simulink model "ssc_vent_splitter_electrical_seriesbag_arch"  (R2020a)
settings: Solver=VariableStepAuto  StartTime=0.0  StopTime=10.0  RelTol=1e-3
settings Model: Creator=jsolislemus  LastModifiedBy=jsolislemus

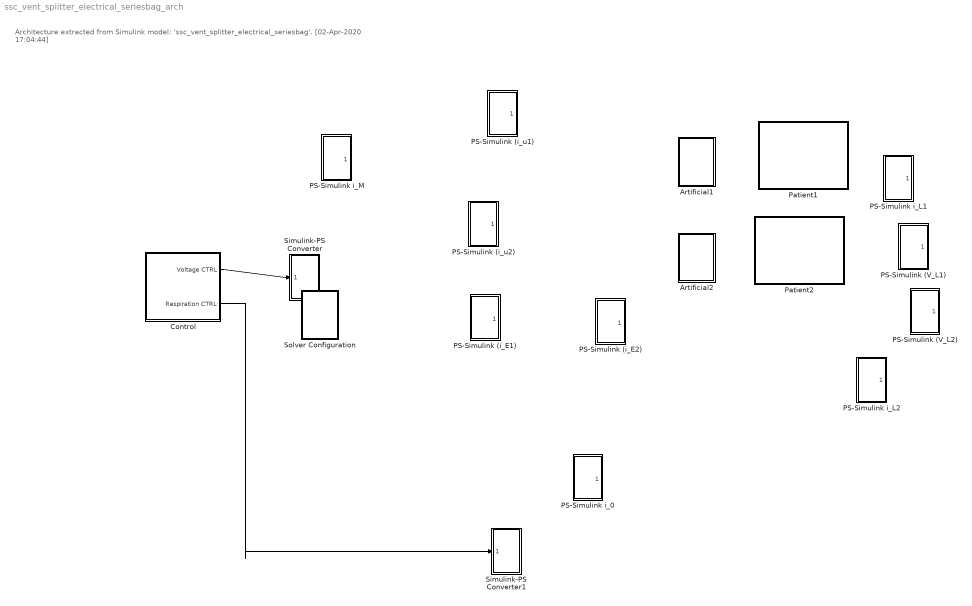
== system ssc_vent_splitter_electrical_seriesbag_arch ==
  note: Architecture extracted from Simulink model: 'ssc_vent_splitter_electrical_seriesbag'. [02-Apr-2020 17:04:44]
  Artificial1 : Subsystem
      settings: PortSchema="{\"entries\":[{\"content\":{\"headerSize\":26,\"margin\":15,\"minimumSpacing\":25,\"sides\":[{\"content\":{\"connectorIds\":[]},\"type\":\"ConnectorPlacement.EquallySpacedRectSide\",\"uuid\":\"6e29aa07-6d05-406a-a3ec-411c5a5a6d59\"},{\"content\":{\"connectorIds\":[],\"side\":\"RIGHT\"},\"type\":\"ConnectorPlacement.EquallySpacedRectSide\",\"uuid\":\"880d3d42-795d-48a8-b736-07df68c99583\"},{\"content\":{\"connectorIds\":[],\"side\":\"TOP\"},\"type\":\"ConnectorPlacement.EquallySpacedRectSide\",\"uuid\":\"00af69ac-1a44-4698-9ec4-d9939426b1cd\"}]},\"type\":\"ConnectorPlacement.EquallySpacedConnector\",\"uuid\":\"8adbbd94-ea7f-44e1-905b-8cd3d9e7fadd\"}],\"packageUris\":[\"http://schema.mathworks.com/mf0/Connector/19700101\"],\"version\":\"1.0\"}"
  Artificial2 : Subsystem
      settings: PortSchema="{\"entries\":[{\"content\":{\"headerSize\":26,\"margin\":15,\"minimumSpacing\":25,\"sides\":[{\"content\":{\"connectorIds\":[]},\"type\":\"ConnectorPlacement.EquallySpacedRectSide\",\"uuid\":\"6e29aa07-6d05-406a-a3ec-411c5a5a6d59\"},{\"content\":{\"connectorIds\":[],\"side\":\"RIGHT\"},\"type\":\"ConnectorPlacement.EquallySpacedRectSide\",\"uuid\":\"880d3d42-795d-48a8-b736-07df68c99583\"},{\"content\":{\"connectorIds\":[],\"side\":\"TOP\"},\"type\":\"ConnectorPlacement.EquallySpacedRectSide\",\"uuid\":\"00af69ac-1a44-4698-9ec4-d9939426b1cd\"}]},\"type\":\"ConnectorPlacement.EquallySpacedConnector\",\"uuid\":\"8adbbd94-ea7f-44e1-905b-8cd3d9e7fadd\"}],\"packageUris\":[\"http://schema.mathworks.com/mf0/Connector/19700101\"],\"version\":\"1.0\"}"
  Control : Subsystem
      settings: PortSchema="{\"entries\":[{\"content\":{\"headerSize\":26,\"margin\":15,\"minimumSpacing\":25,\"sides\":[{\"content\":{\"connectorIds\":[]},\"type\":\"ConnectorPlacement.EquallySpacedRectSide\",\"uuid\":\"868cd02f-3873-4bc0-ad03-13679f5ae2c1\"},{\"content\":{\"connectorIds\":[\"Out1\",\"Out2\"],\"side\":\"RIGHT\"},\"type\":\"ConnectorPlacement.EquallySpacedRectSide\",\"uuid\":\"69928d49-2df3-460f-9e90-f50f969c914b\"},{\"content\":{\"connectorIds\":[],\"side\":\"TOP\"},\"type\":\"ConnectorPlacement.EquallySpacedRectSide\",\"uuid\":\"e58060e5-3c0a-4db3-b34f-65b9832dbc59\"}]},\"type\":\"ConnectorPlacement.EquallySpacedConnector\",\"uuid\":\"a075824f-9c8d-4394-bddd-e7a18dd1991b\"}],\"packageUris\":[\"http://schema.mathworks.com/mf0/Connector/19700101\"],\"version\":\"1.0\"}"
  PS-Simulink (V_L1) : Subsystem
      settings: PortSchema="{\"entries\":[{\"content\":{\"headerSize\":26,\"margin\":15,\"minimumSpacing\":25,\"sides\":[{\"content\":{\"connectorIds\":[]},\"type\":\"ConnectorPlacement.EquallySpacedRectSide\",\"uuid\":\"868cd02f-3873-4bc0-ad03-13679f5ae2c1\"},{\"content\":{\"connectorIds\":[\"Out1\"],\"side\":\"RIGHT\"},\"type\":\"ConnectorPlacement.EquallySpacedRectSide\",\"uuid\":\"69928d49-2df3-460f-9e90-f50f969c914b\"},{\"content\":{\"connectorIds\":[],\"side\":\"TOP\"},\"type\":\"ConnectorPlacement.EquallySpacedRectSide\",\"uuid\":\"e58060e5-3c0a-4db3-b34f-65b9832dbc59\"}]},\"type\":\"ConnectorPlacement.EquallySpacedConnector\",\"uuid\":\"a075824f-9c8d-4394-bddd-e7a18dd1991b\"}],\"packageUris\":[\"http://schema.mathworks.com/mf0/Connector/19700101\"],\"version\":\"1.0\"}"
  PS-Simulink (V_L2) : Subsystem
      settings: PortSchema="{\"entries\":[{\"content\":{\"headerSize\":26,\"margin\":15,\"minimumSpacing\":25,\"sides\":[{\"content\":{\"connectorIds\":[]},\"type\":\"ConnectorPlacement.EquallySpacedRectSide\",\"uuid\":\"868cd02f-3873-4bc0-ad03-13679f5ae2c1\"},{\"content\":{\"connectorIds\":[\"Out1\"],\"side\":\"RIGHT\"},\"type\":\"ConnectorPlacement.EquallySpacedRectSide\",\"uuid\":\"69928d49-2df3-460f-9e90-f50f969c914b\"},{\"content\":{\"connectorIds\":[],\"side\":\"TOP\"},\"type\":\"ConnectorPlacement.EquallySpacedRectSide\",\"uuid\":\"e58060e5-3c0a-4db3-b34f-65b9832dbc59\"}]},\"type\":\"ConnectorPlacement.EquallySpacedConnector\",\"uuid\":\"a075824f-9c8d-4394-bddd-e7a18dd1991b\"}],\"packageUris\":[\"http://schema.mathworks.com/mf0/Connector/19700101\"],\"version\":\"1.0\"}"
  PS-Simulink (i_E1) : Subsystem
      settings: PortSchema="{\"entries\":[{\"content\":{\"headerSize\":26,\"margin\":15,\"minimumSpacing\":25,\"sides\":[{\"content\":{\"connectorIds\":[]},\"type\":\"ConnectorPlacement.EquallySpacedRectSide\",\"uuid\":\"868cd02f-3873-4bc0-ad03-13679f5ae2c1\"},{\"content\":{\"connectorIds\":[\"Out1\"],\"side\":\"RIGHT\"},\"type\":\"ConnectorPlacement.EquallySpacedRectSide\",\"uuid\":\"69928d49-2df3-460f-9e90-f50f969c914b\"},{\"content\":{\"connectorIds\":[],\"side\":\"TOP\"},\"type\":\"ConnectorPlacement.EquallySpacedRectSide\",\"uuid\":\"e58060e5-3c0a-4db3-b34f-65b9832dbc59\"}]},\"type\":\"ConnectorPlacement.EquallySpacedConnector\",\"uuid\":\"a075824f-9c8d-4394-bddd-e7a18dd1991b\"}],\"packageUris\":[\"http://schema.mathworks.com/mf0/Connector/19700101\"],\"version\":\"1.0\"}"
  PS-Simulink (i_E2) : Subsystem
      settings: PortSchema="{\"entries\":[{\"content\":{\"headerSize\":26,\"margin\":15,\"minimumSpacing\":25,\"sides\":[{\"content\":{\"connectorIds\":[]},\"type\":\"ConnectorPlacement.EquallySpacedRectSide\",\"uuid\":\"868cd02f-3873-4bc0-ad03-13679f5ae2c1\"},{\"content\":{\"connectorIds\":[\"Out1\"],\"side\":\"RIGHT\"},\"type\":\"ConnectorPlacement.EquallySpacedRectSide\",\"uuid\":\"69928d49-2df3-460f-9e90-f50f969c914b\"},{\"content\":{\"connectorIds\":[],\"side\":\"TOP\"},\"type\":\"ConnectorPlacement.EquallySpacedRectSide\",\"uuid\":\"e58060e5-3c0a-4db3-b34f-65b9832dbc59\"}]},\"type\":\"ConnectorPlacement.EquallySpacedConnector\",\"uuid\":\"a075824f-9c8d-4394-bddd-e7a18dd1991b\"}],\"packageUris\":[\"http://schema.mathworks.com/mf0/Connector/19700101\"],\"version\":\"1.0\"}"
  PS-Simulink (i_u1) : Subsystem
      settings: PortSchema="{\"entries\":[{\"content\":{\"headerSize\":26,\"margin\":15,\"minimumSpacing\":25,\"sides\":[{\"content\":{\"connectorIds\":[]},\"type\":\"ConnectorPlacement.EquallySpacedRectSide\",\"uuid\":\"868cd02f-3873-4bc0-ad03-13679f5ae2c1\"},{\"content\":{\"connectorIds\":[\"Out1\"],\"side\":\"RIGHT\"},\"type\":\"ConnectorPlacement.EquallySpacedRectSide\",\"uuid\":\"69928d49-2df3-460f-9e90-f50f969c914b\"},{\"content\":{\"connectorIds\":[],\"side\":\"TOP\"},\"type\":\"ConnectorPlacement.EquallySpacedRectSide\",\"uuid\":\"e58060e5-3c0a-4db3-b34f-65b9832dbc59\"}]},\"type\":\"ConnectorPlacement.EquallySpacedConnector\",\"uuid\":\"a075824f-9c8d-4394-bddd-e7a18dd1991b\"}],\"packageUris\":[\"http://schema.mathworks.com/mf0/Connector/19700101\"],\"version\":\"1.0\"}"
  PS-Simulink (i_u2) : Subsystem
      settings: PortSchema="{\"entries\":[{\"content\":{\"headerSize\":26,\"margin\":15,\"minimumSpacing\":25,\"sides\":[{\"content\":{\"connectorIds\":[]},\"type\":\"ConnectorPlacement.EquallySpacedRectSide\",\"uuid\":\"868cd02f-3873-4bc0-ad03-13679f5ae2c1\"},{\"content\":{\"connectorIds\":[\"Out1\"],\"side\":\"RIGHT\"},\"type\":\"ConnectorPlacement.EquallySpacedRectSide\",\"uuid\":\"69928d49-2df3-460f-9e90-f50f969c914b\"},{\"content\":{\"connectorIds\":[],\"side\":\"TOP\"},\"type\":\"ConnectorPlacement.EquallySpacedRectSide\",\"uuid\":\"e58060e5-3c0a-4db3-b34f-65b9832dbc59\"}]},\"type\":\"ConnectorPlacement.EquallySpacedConnector\",\"uuid\":\"a075824f-9c8d-4394-bddd-e7a18dd1991b\"}],\"packageUris\":[\"http://schema.mathworks.com/mf0/Connector/19700101\"],\"version\":\"1.0\"}"
  PS-Simulink i_0 : Subsystem
      settings: PortSchema="{\"entries\":[{\"content\":{\"headerSize\":26,\"margin\":15,\"minimumSpacing\":25,\"sides\":[{\"content\":{\"connectorIds\":[]},\"type\":\"ConnectorPlacement.EquallySpacedRectSide\",\"uuid\":\"868cd02f-3873-4bc0-ad03-13679f5ae2c1\"},{\"content\":{\"connectorIds\":[\"Out1\"],\"side\":\"RIGHT\"},\"type\":\"ConnectorPlacement.EquallySpacedRectSide\",\"uuid\":\"69928d49-2df3-460f-9e90-f50f969c914b\"},{\"content\":{\"connectorIds\":[],\"side\":\"TOP\"},\"type\":\"ConnectorPlacement.EquallySpacedRectSide\",\"uuid\":\"e58060e5-3c0a-4db3-b34f-65b9832dbc59\"}]},\"type\":\"ConnectorPlacement.EquallySpacedConnector\",\"uuid\":\"a075824f-9c8d-4394-bddd-e7a18dd1991b\"}],\"packageUris\":[\"http://schema.mathworks.com/mf0/Connector/19700101\"],\"version\":\"1.0\"}"
  PS-Simulink i_L1 : Subsystem
      settings: PortSchema="{\"entries\":[{\"content\":{\"headerSize\":26,\"margin\":15,\"minimumSpacing\":25,\"sides\":[{\"content\":{\"connectorIds\":[]},\"type\":\"ConnectorPlacement.EquallySpacedRectSide\",\"uuid\":\"868cd02f-3873-4bc0-ad03-13679f5ae2c1\"},{\"content\":{\"connectorIds\":[\"Out1\"],\"side\":\"RIGHT\"},\"type\":\"ConnectorPlacement.EquallySpacedRectSide\",\"uuid\":\"69928d49-2df3-460f-9e90-f50f969c914b\"},{\"content\":{\"connectorIds\":[],\"side\":\"TOP\"},\"type\":\"ConnectorPlacement.EquallySpacedRectSide\",\"uuid\":\"e58060e5-3c0a-4db3-b34f-65b9832dbc59\"}]},\"type\":\"ConnectorPlacement.EquallySpacedConnector\",\"uuid\":\"a075824f-9c8d-4394-bddd-e7a18dd1991b\"}],\"packageUris\":[\"http://schema.mathworks.com/mf0/Connector/19700101\"],\"version\":\"1.0\"}"
  PS-Simulink i_L2 : Subsystem
      settings: PortSchema="{\"entries\":[{\"content\":{\"headerSize\":26,\"margin\":15,\"minimumSpacing\":25,\"sides\":[{\"content\":{\"connectorIds\":[]},\"type\":\"ConnectorPlacement.EquallySpacedRectSide\",\"uuid\":\"868cd02f-3873-4bc0-ad03-13679f5ae2c1\"},{\"content\":{\"connectorIds\":[\"Out1\"],\"side\":\"RIGHT\"},\"type\":\"ConnectorPlacement.EquallySpacedRectSide\",\"uuid\":\"69928d49-2df3-460f-9e90-f50f969c914b\"},{\"content\":{\"connectorIds\":[],\"side\":\"TOP\"},\"type\":\"ConnectorPlacement.EquallySpacedRectSide\",\"uuid\":\"e58060e5-3c0a-4db3-b34f-65b9832dbc59\"}]},\"type\":\"ConnectorPlacement.EquallySpacedConnector\",\"uuid\":\"a075824f-9c8d-4394-bddd-e7a18dd1991b\"}],\"packageUris\":[\"http://schema.mathworks.com/mf0/Connector/19700101\"],\"version\":\"1.0\"}"
  PS-Simulink i_M : Subsystem
      settings: PortSchema="{\"entries\":[{\"content\":{\"headerSize\":26,\"margin\":15,\"minimumSpacing\":25,\"sides\":[{\"content\":{\"connectorIds\":[]},\"type\":\"ConnectorPlacement.EquallySpacedRectSide\",\"uuid\":\"868cd02f-3873-4bc0-ad03-13679f5ae2c1\"},{\"content\":{\"connectorIds\":[\"Out1\"],\"side\":\"RIGHT\"},\"type\":\"ConnectorPlacement.EquallySpacedRectSide\",\"uuid\":\"69928d49-2df3-460f-9e90-f50f969c914b\"},{\"content\":{\"connectorIds\":[],\"side\":\"TOP\"},\"type\":\"ConnectorPlacement.EquallySpacedRectSide\",\"uuid\":\"e58060e5-3c0a-4db3-b34f-65b9832dbc59\"}]},\"type\":\"ConnectorPlacement.EquallySpacedConnector\",\"uuid\":\"a075824f-9c8d-4394-bddd-e7a18dd1991b\"}],\"packageUris\":[\"http://schema.mathworks.com/mf0/Connector/19700101\"],\"version\":\"1.0\"}"
  Patient1 : Subsystem
      settings: PortSchema="{\"entries\":[{\"content\":{\"headerSize\":26,\"margin\":15,\"minimumSpacing\":25,\"sides\":[{\"content\":{\"connectorIds\":[]},\"type\":\"ConnectorPlacement.EquallySpacedRectSide\",\"uuid\":\"6e29aa07-6d05-406a-a3ec-411c5a5a6d59\"},{\"content\":{\"connectorIds\":[],\"side\":\"RIGHT\"},\"type\":\"ConnectorPlacement.EquallySpacedRectSide\",\"uuid\":\"880d3d42-795d-48a8-b736-07df68c99583\"},{\"content\":{\"connectorIds\":[],\"side\":\"TOP\"},\"type\":\"ConnectorPlacement.EquallySpacedRectSide\",\"uuid\":\"00af69ac-1a44-4698-9ec4-d9939426b1cd\"}]},\"type\":\"ConnectorPlacement.EquallySpacedConnector\",\"uuid\":\"8adbbd94-ea7f-44e1-905b-8cd3d9e7fadd\"}],\"packageUris\":[\"http://schema.mathworks.com/mf0/Connector/19700101\"],\"version\":\"1.0\"}"
  Patient2 : Subsystem
      settings: PortSchema="{\"entries\":[{\"content\":{\"headerSize\":26,\"margin\":15,\"minimumSpacing\":25,\"sides\":[{\"content\":{\"connectorIds\":[]},\"type\":\"ConnectorPlacement.EquallySpacedRectSide\",\"uuid\":\"6e29aa07-6d05-406a-a3ec-411c5a5a6d59\"},{\"content\":{\"connectorIds\":[],\"side\":\"RIGHT\"},\"type\":\"ConnectorPlacement.EquallySpacedRectSide\",\"uuid\":\"880d3d42-795d-48a8-b736-07df68c99583\"},{\"content\":{\"connectorIds\":[],\"side\":\"TOP\"},\"type\":\"ConnectorPlacement.EquallySpacedRectSide\",\"uuid\":\"00af69ac-1a44-4698-9ec4-d9939426b1cd\"}]},\"type\":\"ConnectorPlacement.EquallySpacedConnector\",\"uuid\":\"8adbbd94-ea7f-44e1-905b-8cd3d9e7fadd\"}],\"packageUris\":[\"http://schema.mathworks.com/mf0/Connector/19700101\"],\"version\":\"1.0\"}"
  Simulink-PS Converter : Subsystem
      settings: PortSchema="{\"entries\":[{\"content\":{\"headerSize\":26,\"margin\":15,\"minimumSpacing\":25,\"sides\":[{\"content\":{\"connectorIds\":[\"In1\"]},\"type\":\"ConnectorPlacement.EquallySpacedRectSide\",\"uuid\":\"5530b401-d909-4278-b452-8be52398f419\"},{\"content\":{\"connectorIds\":[],\"side\":\"RIGHT\"},\"type\":\"ConnectorPlacement.EquallySpacedRectSide\",\"uuid\":\"b30f23cc-90a7-4a08-a36d-4f9e93885a54\"},{\"content\":{\"connectorIds\":[],\"side\":\"TOP\"},\"type\":\"ConnectorPlacement.EquallySpacedRectSide\",\"uuid\":\"2eed8453-9701-4d20-adee-7c5c4b98195e\"}]},\"type\":\"ConnectorPlacement.EquallySpacedConnector\",\"uuid\":\"41ee2832-6870-428c-ad87-eb5e13e130a4\"}],\"packageUris\":[\"http://schema.mathworks.com/mf0/Connector/19700101\"],\"version\":\"1.0\"}"
  Simulink-PS Converter1 : Subsystem
      settings: PortSchema="{\"entries\":[{\"content\":{\"headerSize\":26,\"margin\":15,\"minimumSpacing\":25,\"sides\":[{\"content\":{\"connectorIds\":[\"In1\"]},\"type\":\"ConnectorPlacement.EquallySpacedRectSide\",\"uuid\":\"5530b401-d909-4278-b452-8be52398f419\"},{\"content\":{\"connectorIds\":[],\"side\":\"RIGHT\"},\"type\":\"ConnectorPlacement.EquallySpacedRectSide\",\"uuid\":\"b30f23cc-90a7-4a08-a36d-4f9e93885a54\"},{\"content\":{\"connectorIds\":[],\"side\":\"TOP\"},\"type\":\"ConnectorPlacement.EquallySpacedRectSide\",\"uuid\":\"2eed8453-9701-4d20-adee-7c5c4b98195e\"}]},\"type\":\"ConnectorPlacement.EquallySpacedConnector\",\"uuid\":\"41ee2832-6870-428c-ad87-eb5e13e130a4\"}],\"packageUris\":[\"http://schema.mathworks.com/mf0/Connector/19700101\"],\"version\":\"1.0\"}"
  Solver Configuration : Subsystem
      settings: PortSchema="{\"entries\":[{\"content\":{\"headerSize\":26,\"margin\":15,\"minimumSpacing\":25,\"sides\":[{\"content\":{\"connectorIds\":[]},\"type\":\"ConnectorPlacement.EquallySpacedRectSide\",\"uuid\":\"6e29aa07-6d05-406a-a3ec-411c5a5a6d59\"},{\"content\":{\"connectorIds\":[],\"side\":\"RIGHT\"},\"type\":\"ConnectorPlacement.EquallySpacedRectSide\",\"uuid\":\"880d3d42-795d-48a8-b736-07df68c99583\"},{\"content\":{\"connectorIds\":[],\"side\":\"TOP\"},\"type\":\"ConnectorPlacement.EquallySpacedRectSide\",\"uuid\":\"00af69ac-1a44-4698-9ec4-d9939426b1cd\"}]},\"type\":\"ConnectorPlacement.EquallySpacedConnector\",\"uuid\":\"8adbbd94-ea7f-44e1-905b-8cd3d9e7fadd\"}],\"packageUris\":[\"http://schema.mathworks.com/mf0/Connector/19700101\"],\"version\":\"1.0\"}"
  wires:
  Control/1(Voltage CTRL) -> Simulink-PS Converter/1(input0)
  Control/2(Respiration CTRL) -> Simulink-PS Converter1/1(input0)

== system ssc_vent_splitter_electrical_seriesbag_arch/Artificial1 ==

== system ssc_vent_splitter_electrical_seriesbag_arch/Artificial2 ==

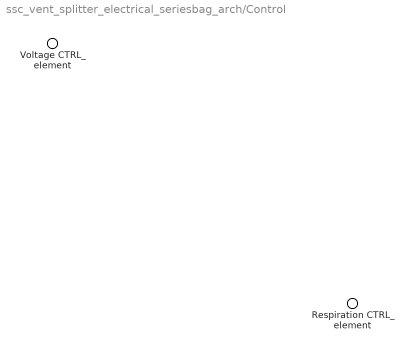
== system ssc_vent_splitter_electrical_seriesbag_arch/Control ==
  Voltage CTRL_element : Outport  PortName=Voltage CTRL
  Respiration CTRL_element : Outport  Port=2  PortName=Respiration CTRL

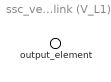
== system ssc_vent_splitter_electrical_seriesbag_arch/PS-Simulink (V_L1) ==
  output_element : Outport  PortName=output

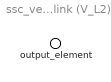
== system ssc_vent_splitter_electrical_seriesbag_arch/PS-Simulink (V_L2) ==
  output_element : Outport  PortName=output

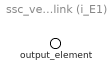
== system ssc_vent_splitter_electrical_seriesbag_arch/PS-Simulink (i_E1) ==
  output_element : Outport  PortName=output

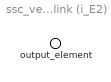
== system ssc_vent_splitter_electrical_seriesbag_arch/PS-Simulink (i_E2) ==
  output_element : Outport  PortName=output

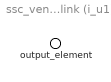
== system ssc_vent_splitter_electrical_seriesbag_arch/PS-Simulink (i_u1) ==
  output_element : Outport  PortName=output

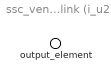
== system ssc_vent_splitter_electrical_seriesbag_arch/PS-Simulink (i_u2) ==
  output_element : Outport  PortName=output

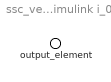
== system ssc_vent_splitter_electrical_seriesbag_arch/PS-Simulink i_0 ==
  output_element : Outport  PortName=output

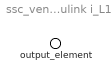
== system ssc_vent_splitter_electrical_seriesbag_arch/PS-Simulink i_L1 ==
  output_element : Outport  PortName=output

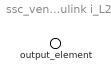
== system ssc_vent_splitter_electrical_seriesbag_arch/PS-Simulink i_L2 ==
  output_element : Outport  PortName=output

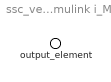
== system ssc_vent_splitter_electrical_seriesbag_arch/PS-Simulink i_M ==
  output_element : Outport  PortName=output

== system ssc_vent_splitter_electrical_seriesbag_arch/Patient1 ==

== system ssc_vent_splitter_electrical_seriesbag_arch/Patient2 ==

== system ssc_vent_splitter_electrical_seriesbag_arch/Simulink-PS Converter ==
  input0_element : Inport  PortName=input0

== system ssc_vent_splitter_electrical_seriesbag_arch/Simulink-PS Converter1 ==
  input0_element : Inport  PortName=input0

== system ssc_vent_splitter_electrical_seriesbag_arch/Solver Configuration ==
